simulink model "untitled"  (R2013b)
settings: Solver=ode3  StartTime=0.0  StopTime=10.0  FixedStep=0.02  RelTol=1e-3
libraries: simulink x1
settings Model: Creator=Eduardo  LastModifiedBy=Eduardo
settings OptimizationCC: OptimizeModelRefInitCode=on  LifeSpan=1
settings RTWCC: SystemTargetFile=ert.tlc  TemplateMakefile=ert_default_tmf  Description=Embedded Coder  ProcessScript=ert_make_rtw_hook
settings CodeAppCC: IgnoreCustomStorageClasses=off
settings ERTTargetCC: CodeReplacementLibrary=ANSI_C  GenerateSampleERTMain=on  ERTCustomFileTemplate=example_file_process.tlc

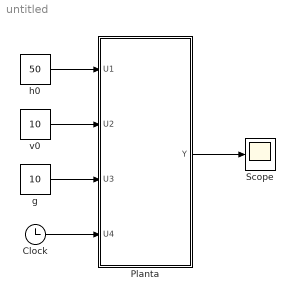
== system untitled ==
  Clock : Clock
  Planta : Subsystem
  Scope : Scope
  g : Constant  Value=10
  h0 : Constant  Value=50
  "v0 " : Constant  Value=10
  wires:
  h0/1 -> Planta/1(U1)
  "v0 "/1 -> Planta/2(U2)
  g/1 -> Planta/3(U3)
  Clock/1 -> Planta/4(U4)
  Planta/1(Y) -> Scope/1

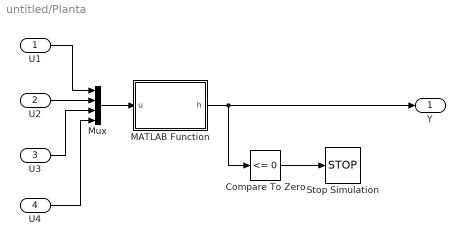
== system untitled/Planta ==
  U1 : Inport
  U2 : Inport  Port=2
  U3 : Inport  Port=3
  U4 : Inport  Port=4
  Compare To Zero : simulink/Logic and Bit Operations/Compare To Zero  relop=<=  OutDataTypeStr=boolean
  MATLAB Function : MATLAB Function  TreatAsAtomicUnit=on
  Mux : Mux
  Stop Simulation : Stop
  Y : Outport
  wires:
  MATLAB Function/1(h) -> Y/1, Compare To Zero/1
  Compare To Zero/1 -> Stop Simulation/1
  Mux/1 -> MATLAB Function/1(u)
  U1/1 -> Mux/1
  U3/1 -> Mux/3
  U2/1 -> Mux/2
  U4/1 -> Mux/4

== matlab function untitled/Planta/MATLAB Function ==
  data: u input; h output
function h = fcn(u)

% Pega as entradas.
h0 = u(1);
v0 = u(2);
g  = u(3);
t  = u(4);

% Calcula a altura.
h = h0 + v0*t - 0.5*g*t^2;
